simulink model "simulink_1"  (R2017b)
settings: Solver=VariableStepAuto  StartTime=0.0  StopTime=10  MaxStep=1e-5  RelTol=1e-3
libraries: rfmathmodels1 x2
settings Model: Creator=bocheng  LastModifiedBy=bocheng

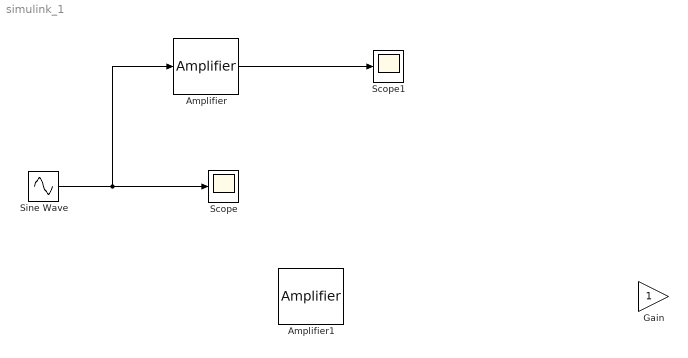
== system simulink_1 ==
  Amplifier : rfmathmodels1/Amplifier  model_select=Linear  linGaindB=1  GindB=0  iip3=30  am2pm=10  PwrAMPMStart=10  PwrAMPMEnd=inf  amam=[2.1587 1.1517]  ampm=[4.0033 9.1040]  x=[8.1081 1.5413 6.5202 -0.0718]  y=[4.6645 2.0965 10.88 -0.003]  p=0.5  GoutdB=0  vsat=1  method_select=Noise factor  ntemp=290  nfigure=3.01  nfactor=2  seed=67987
      settings: SourceProductName=RF Toolbox  SourceProductBaseCode=RF
  Amplifier1 : rfmathmodels1/Amplifier  model_select=Linear  linGaindB=1  GindB=0  iip3=30  am2pm=10  PwrAMPMStart=10  PwrAMPMEnd=inf  amam=[2.1587 1.1517]  ampm=[4.0033 9.1040]  x=[8.1081 1.5413 6.5202 -0.0718]  y=[4.6645 2.0965 10.88 -0.003]  p=0.5  GoutdB=0  vsat=1  method_select=Noise factor  ntemp=290  nfigure=3.01  nfactor=2  seed=67987
      settings: SourceProductName=RF Toolbox  SourceProductBaseCode=RF
  Gain : Gain
  Scope : Scope
  Scope1 : Scope
  Sine Wave : Sin  Frequency=200*pi  SampleTime=0
  wires:
  Sine Wave/1 -> Amplifier/1, Scope/1
  Amplifier/1 -> Scope1/1
